simulink model "simple_MAV_Simulink"  (R2019a)
settings: Solver=ode4  StartTime=0.0  StopTime=50  FixedStep=P.Ts  RelTol=1e-3
libraries: simulink x1
settings Model: Creator=simao  LastModifiedBy=simao

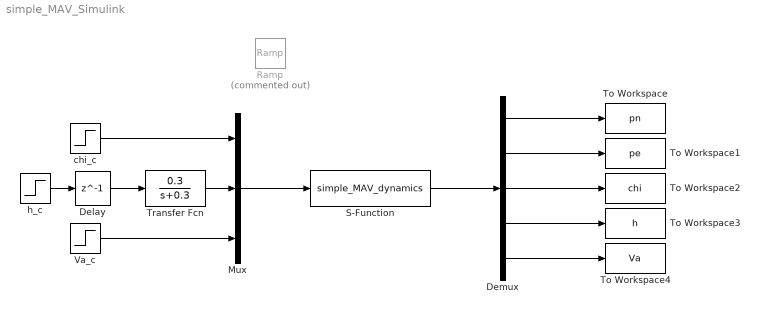
== system simple_MAV_Simulink ==
  Delay : Delay  DelayLength=1  SampleTime=1
  Demux : Demux  Outputs=5
  Mux : Mux  Inputs=3
  Ramp : simulink/Sources/Ramp  Commented=on  slope=0.5  start=0  InitialOutput=0
  S-Function : S-Function  FunctionName=simple_MAV_dynamics  Parameters=P  SFunctionDeploymentMode=off  EnableBusSupport=off
  To Workspace : ToWorkspace  VariableName=pn  SaveFormat=Timeseries  SampleTime=-1
  To Workspace1 : ToWorkspace  VariableName=pe  SaveFormat=Timeseries  SampleTime=-1
  To Workspace2 : ToWorkspace  VariableName=chi  SaveFormat=Timeseries  SampleTime=-1
  To Workspace3 : ToWorkspace  VariableName=h  SaveFormat=Timeseries  SampleTime=-1
  To Workspace4 : ToWorkspace  VariableName=Va  SaveFormat=Timeseries  SampleTime=-1
  Transfer Fcn : TransferFcn  Numerator=[0.3]  Denominator=[1 0.3]
  Va_c : Step  Time=0  After=30  SampleTime=0
  chi_c : Step  Time=0  After=10*pi/180  SampleTime=0
  h_c : Step  Time=0  After=200  SampleTime=0
  wires:
  Demux/1 -> To Workspace/1
  Demux/2 -> To Workspace1/1
  Demux/3 -> To Workspace2/1
  Demux/5 -> To Workspace4/1
  Demux/4 -> To Workspace3/1
  Mux/1 -> S-Function/1
  S-Function/1 -> Demux/1
  Va_c/1 -> Mux/3
  chi_c/1 -> Mux/1
  h_c/1 -> Delay/1
  Delay/1 -> Transfer Fcn/1
  Transfer Fcn/1 -> Mux/2
